simulink model "Torque Vectoring and Ackerman Model"  (R2020b)
settings: Solver=ode4  StartTime=0.0  StopTime=12  FixedStep=1e-5  RelTol=1e-3
InitFcn:
  | clc
  | clear
  | clc;
  | clear;
  | Ts=1e-5; %Sampling time
  | f=50; %Supply frequency
  | Rs=0.03553; %Stator resistance
  | Rr=0.02092; %Rotor resistance
  | Lls=0.000335; %Stator inductance
  | Llr=0.000335; %Rotor inductance
  | Lm=0.0151; %Mutual inductance
  | P=4; %Number of Poles
  | ts=(Lls+Lm)/Rs; % Stator time constant
  | Tr=(Llr+Lm)/Rr; % Rotor time constant
  | Ls=Lls+Lm;
  | Lrr=Llr+Lm;
  | J=1.25; %Inertia
  | F=0.03914; %Friction factor
  | VDC=580;
  | sigma=1-(Lm^2/(Ls*Lrr));
  | rs=Rs+Rr*(Lm/Lrr)^2;
  | Kp=1498*sigma*Ls;
  | Ki=rs*1498;
  | dw=1.55;
  | l=3;
  | m       =       1500;           %Vehicle mass
  | g       =       9.81;           %Gravitational acceleration
  | L       =          3;           %Distance between front axle and rear axle
  | Lf      =        1.3;           %Distance between center of mass and front axle
  | Lr      =       L-Lf;           %Distance between center of mass and rear axle
  | Cf      =      67369;           %Front track Cornering stiffness coef
  | Cr      =      63411;           %rear track Cornering stiffness coef
  | S       =        1.7;           %Area of frontal surface of the vehicle
  | CYB     =       -2.2;           %Force drag coef
  | CMzB    =        0.6;           %Moment drag coef
  | Mzfa    =       2010;           %Front track Aligning stiffness coef
  | Mzra    =       1366;           %rear track Aligning stiffness coef
  | rho     =      1.225;           %density
  | Iz      =       2000;           %Yaw Moment of Inertia
  | Kgear=1;
undefined symbols (not defined in the file): DiscIntNeverNeededParam, Driver, Wheels_Driver_VehDyn_Lib
libraries: pid_lib x12, powerlib_meascontrol x11, powerlib x9, simulink_extras x4
(part 2 of 2)

== system Torque Vectoring and Ackerman Model/Right Motor/FOC1/Vd ==
  Phir* : Inport
  id : Inport  Port=2
  Current PI : pid_lib/PID Controller  Controller=PI  Form=Parallel  TimeDomain=Discrete-time  UseExternalTs=off  SampleTime=Ts  IntegratorMethod=Forward Euler  FilterMethod=Forward Euler  ControllerParametersSource=internal  P=Kp  I=Ki  D=0  UseFilter=on  N=100  TunerSelectOption=Transfer Function Based (PID Tuner App)  InitialConditionSource=internal  InitialConditionForIntegrator=0  InitialConditionForFilter=0  DifferentiatorICPrevScaledInput=0  ExternalReset=none  TrackingMode=off  Kt=1  LimitOutput=on  SatLimitsSource=internal  UpperSaturationLimit=VDC  LowerSaturationLimit=-VDC/2  LinearizeAsGain=off  AntiWindupMode=clamping  Kb=1  POutMin=[]  POutMax=[]  IOutMin=[]  IOutMax=[]  DOutMin=[]  DOutMax=[]  NOutMin=[]  NOutMax=[]  SumOutMin=[]  SumOutMax=[]  SaturationOutMin=[]  SaturationOutMax=[]  PParamMin=[]  PParamMax=[]  IParamMin=[]  IParamMax=[]  DParamMin=[]  DParamMax=[]  NParamMin=[]  NParamMax=[]  KbParamMin=[]  KbParamMax=[]  KtParamMin=[]  KtParamMax=[]  KbOutMin=[]  KbOutMax=[]  KtOutMin=[]  KtOutMax=[]  IntegratorOutMin=[]  IntegratorOutMax=[]  FilterOutMin=[]  FilterOutMax=[]  SumI1OutMin=[]  SumI1OutMax=[]  SumI2OutMin=[]  SumI2OutMax=[]  SumI3OutMin=[]  SumI3OutMax=[]  SumI4OutMin=[]  SumI4OutMax=[]  SumDOutMin=[]  SumDOutMax=[]  DifferentiatorOutMin=[]  DifferentiatorOutMax=[]  FilterDiffOutCoefMin=[]  FilterDiffOutCoefMax=[]  ReciprocalOutMin=[]  ReciprocalOutMax=[]  SumDenOutMin=[]  SumDenOutMax=[]  SumNumOutMin=[]  SumNumOutMax=[]  DivideOutMin=[]  DivideOutMax=[]  UdiffTsProdOutMin=[]  UdiffTsProdOutMax=[]  NTsProdOutMin=[]  NTsProdOutMax=[]  UintegralTsProdOutMin=[]  UintegralTsProdOutMax=[]  UngainTsProdOutMin=[]  UngainTsProdOutMax=[]  IntegratorContinuousStateAttributes=''  IntegratorStateMustResolveToSignalObject=off  IntegratorRTWStateStorageClass=Auto  FilterContinuousStateAttributes=''  FilterStateMustResolveToSignalObject=off  FilterRTWStateStorageClass=Auto  ParallelPVariant=InternalParameters  IdealPVariant=Disabled  IVariant=InternalParameters  DVariant=Disabled  IntegratorVariant=Discrete  SatVariant=Enabled  AWVariant=DiscClampingParallel  PCopyVariant=Disabled  TRVariant=Disabled  FdbkBlocksVariant=Forward  IdealPFdbkVariant=Disabled  SatFdbkVariant=Disabled  DerivativeFilterVariant=Disabled  NVariant=Disabled  NCopyVariant=Disabled_SignalSpec  FilterICVariant=Disabled  IntegratorICVariant=InternalICs  ExternalResetVariant=Disabled  TRSumVariant=Passthrough  SumFdbkVariant=Disabled  SumVariant=Sum_PI  TsampFilterVariant=InternalTs  TsampNgainVariant=Passthrough  TsampIntegralVariant=Passthrough  ExternalSaturationOutDataTypeStr=Inherit: Same as second input
  Gain : Gain  Gain=1/Lm
  Scope : Scope
  Sum2 : Sum  Inputs=|+-
  Vd : Outport
  tag scope: IdrefR=global
  wires:
  Gain/1 -> [IdrefR], Scope/1, Sum2/1
  Phir*/1 -> Gain/1
  id/1 -> Sum2/2
  Sum2/1 -> Current PI/1
  Current PI/1 -> Vd/1

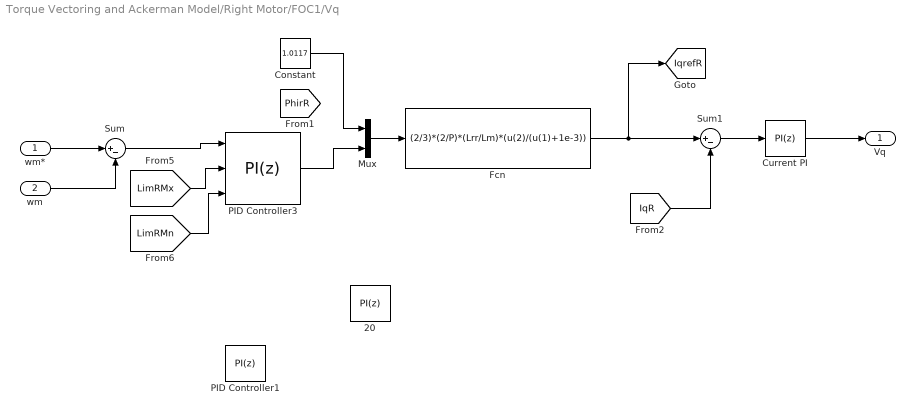
== system Torque Vectoring and Ackerman Model/Right Motor/FOC1/Vq ==
  wm* : Inport
  wm : Inport  Port=2
  20 : pid_lib/PID Controller  Controller=PI  Form=Parallel  TimeDomain=Discrete-time  UseExternalTs=off  SampleTime=-1  IntegratorMethod=Forward Euler  FilterMethod=Forward Euler  ControllerParametersSource=internal  P=152.4390244  I=9295.062463  D=0  UseFilter=on  N=100  TunerSelectOption=Transfer Function Based (PID Tuner App)  InitialConditionSource=internal  InitialConditionForIntegrator=0  InitialConditionForFilter=0  DifferentiatorICPrevScaledInput=0  ExternalReset=none  TrackingMode=off  Kt=1  LimitOutput=on  SatLimitsSource=internal  UpperSaturationLimit=960  LowerSaturationLimit=-960  LinearizeAsGain=off  AntiWindupMode=clamping  Kb=1  POutMin=[]  POutMax=[]  IOutMin=[]  IOutMax=[]  DOutMin=[]  DOutMax=[]  NOutMin=[]  NOutMax=[]  SumOutMin=[]  SumOutMax=[]  SaturationOutMin=[]  SaturationOutMax=[]  PParamMin=[]  PParamMax=[]  IParamMin=[]  IParamMax=[]  DParamMin=[]  DParamMax=[]  NParamMin=[]  NParamMax=[]  KbParamMin=[]  KbParamMax=[]  KtParamMin=[]  KtParamMax=[]  KbOutMin=[]  KbOutMax=[]  KtOutMin=[]  KtOutMax=[]  IntegratorOutMin=[]  IntegratorOutMax=[]  FilterOutMin=[]  FilterOutMax=[]  SumI1OutMin=[]  SumI1OutMax=[]  SumI2OutMin=[]  SumI2OutMax=[]  SumI3OutMin=[]  SumI3OutMax=[]  SumI4OutMin=[]  SumI4OutMax=[]  SumDOutMin=[]  SumDOutMax=[]  DifferentiatorOutMin=[]  DifferentiatorOutMax=[]  FilterDiffOutCoefMin=[]  FilterDiffOutCoefMax=[]  ReciprocalOutMin=[]  ReciprocalOutMax=[]  SumDenOutMin=[]  SumDenOutMax=[]  SumNumOutMin=[]  SumNumOutMax=[]  DivideOutMin=[]  DivideOutMax=[]  UdiffTsProdOutMin=[]  UdiffTsProdOutMax=[]  NTsProdOutMin=[]  NTsProdOutMax=[]  UintegralTsProdOutMin=[]  UintegralTsProdOutMax=[]  UngainTsProdOutMin=[]  UngainTsProdOutMax=[]  IntegratorContinuousStateAttributes=''  IntegratorStateMustResolveToSignalObject=off  IntegratorRTWStateStorageClass=Auto  FilterContinuousStateAttributes=''  FilterStateMustResolveToSignalObject=off  FilterRTWStateStorageClass=Auto  ParallelPVariant=InternalParameters  IdealPVariant=Disabled  IVariant=InternalParameters  DVariant=Disabled  IntegratorVariant=Discrete  SatVariant=Enabled  AWVariant=DiscClampingParallel  PCopyVariant=Disabled  TRVariant=Disabled  FdbkBlocksVariant=Forward  IdealPFdbkVariant=Disabled  SatFdbkVariant=Disabled  DerivativeFilterVariant=Disabled  NVariant=Disabled  NCopyVariant=Disabled_SignalSpec  FilterICVariant=Disabled  IntegratorICVariant=InternalICs  ExternalResetVariant=Disabled  TRSumVariant=Passthrough  SumFdbkVariant=Disabled  SumVariant=Sum_PI  TsampFilterVariant=InternalTs  TsampNgainVariant=Passthrough  TsampIntegralVariant=Passthrough  ExternalSaturationOutDataTypeStr=Inherit: Same as second input
  Constant : Constant  Value=1.0117
  Current PI : pid_lib/PID Controller  Controller=PI  Form=Parallel  TimeDomain=Discrete-time  UseExternalTs=off  SampleTime=Ts  IntegratorMethod=Forward Euler  FilterMethod=Forward Euler  ControllerParametersSource=internal  P=Kp  I=Ki  D=0  UseFilter=on  N=100  TunerSelectOption=Transfer Function Based (PID Tuner App)  InitialConditionSource=internal  InitialConditionForIntegrator=0  InitialConditionForFilter=0  DifferentiatorICPrevScaledInput=0  ExternalReset=none  TrackingMode=off  Kt=1  LimitOutput=on  SatLimitsSource=internal  UpperSaturationLimit=VDC/sqrt(3)  LowerSaturationLimit=-VDC/sqrt(3)  LinearizeAsGain=off  AntiWindupMode=clamping  Kb=1  POutMin=[]  POutMax=[]  IOutMin=[]  IOutMax=[]  DOutMin=[]  DOutMax=[]  NOutMin=[]  NOutMax=[]  SumOutMin=[]  SumOutMax=[]  SaturationOutMin=[]  SaturationOutMax=[]  PParamMin=[]  PParamMax=[]  IParamMin=[]  IParamMax=[]  DParamMin=[]  DParamMax=[]  NParamMin=[]  NParamMax=[]  KbParamMin=[]  KbParamMax=[]  KtParamMin=[]  KtParamMax=[]  KbOutMin=[]  KbOutMax=[]  KtOutMin=[]  KtOutMax=[]  IntegratorOutMin=[]  IntegratorOutMax=[]  FilterOutMin=[]  FilterOutMax=[]  SumI1OutMin=[]  SumI1OutMax=[]  SumI2OutMin=[]  SumI2OutMax=[]  SumI3OutMin=[]  SumI3OutMax=[]  SumI4OutMin=[]  SumI4OutMax=[]  SumDOutMin=[]  SumDOutMax=[]  DifferentiatorOutMin=[]  DifferentiatorOutMax=[]  FilterDiffOutCoefMin=[]  FilterDiffOutCoefMax=[]  ReciprocalOutMin=[]  ReciprocalOutMax=[]  SumDenOutMin=[]  SumDenOutMax=[]  SumNumOutMin=[]  SumNumOutMax=[]  DivideOutMin=[]  DivideOutMax=[]  UdiffTsProdOutMin=[]  UdiffTsProdOutMax=[]  NTsProdOutMin=[]  NTsProdOutMax=[]  UintegralTsProdOutMin=[]  UintegralTsProdOutMax=[]  UngainTsProdOutMin=[]  UngainTsProdOutMax=[]  IntegratorContinuousStateAttributes=''  IntegratorStateMustResolveToSignalObject=off  IntegratorRTWStateStorageClass=Auto  FilterContinuousStateAttributes=''  FilterStateMustResolveToSignalObject=off  FilterRTWStateStorageClass=Auto  ParallelPVariant=InternalParameters  IdealPVariant=Disabled  IVariant=InternalParameters  DVariant=Disabled  IntegratorVariant=Discrete  SatVariant=Enabled  AWVariant=DiscClampingParallel  PCopyVariant=Disabled  TRVariant=Disabled  FdbkBlocksVariant=Forward  IdealPFdbkVariant=Disabled  SatFdbkVariant=Disabled  DerivativeFilterVariant=Disabled  NVariant=Disabled  NCopyVariant=Disabled_SignalSpec  FilterICVariant=Disabled  IntegratorICVariant=InternalICs  ExternalResetVariant=Disabled  TRSumVariant=Passthrough  SumFdbkVariant=Disabled  SumVariant=Sum_PI  TsampFilterVariant=InternalTs  TsampNgainVariant=Passthrough  TsampIntegralVariant=Passthrough  ExternalSaturationOutDataTypeStr=Inherit: Same as second input
  Fcn : Fcn  Expr=(2/3)*(2/P)*(Lrr/Lm)*(u(2)/(u(1)+1e-3))
  Mux : Mux  Inputs=2
  PID Controller1 : pid_lib/PID Controller  Controller=PI  Form=Parallel  TimeDomain=Discrete-time  UseExternalTs=off  SampleTime=-1  IntegratorMethod=Forward Euler  FilterMethod=Forward Euler  ControllerParametersSource=internal  P=105.005210798555  I=869.041988278239  D=0  UseFilter=on  N=100  TunerSelectOption=Transfer Function Based (PID Tuner App)  InitialConditionSource=internal  InitialConditionForIntegrator=0  InitialConditionForFilter=0  DifferentiatorICPrevScaledInput=0  ExternalReset=none  TrackingMode=off  Kt=1  LimitOutput=on  SatLimitsSource=internal  UpperSaturationLimit=960  LowerSaturationLimit=-960  LinearizeAsGain=off  AntiWindupMode=clamping  Kb=1  POutMin=[]  POutMax=[]  IOutMin=[]  IOutMax=[]  DOutMin=[]  DOutMax=[]  NOutMin=[]  NOutMax=[]  SumOutMin=[]  SumOutMax=[]  SaturationOutMin=[]  SaturationOutMax=[]  PParamMin=[]  PParamMax=[]  IParamMin=[]  IParamMax=[]  DParamMin=[]  DParamMax=[]  NParamMin=[]  NParamMax=[]  KbParamMin=[]  KbParamMax=[]  KtParamMin=[]  KtParamMax=[]  KbOutMin=[]  KbOutMax=[]  KtOutMin=[]  KtOutMax=[]  IntegratorOutMin=[]  IntegratorOutMax=[]  FilterOutMin=[]  FilterOutMax=[]  SumI1OutMin=[]  SumI1OutMax=[]  SumI2OutMin=[]  SumI2OutMax=[]  SumI3OutMin=[]  SumI3OutMax=[]  SumI4OutMin=[]  SumI4OutMax=[]  SumDOutMin=[]  SumDOutMax=[]  DifferentiatorOutMin=[]  DifferentiatorOutMax=[]  FilterDiffOutCoefMin=[]  FilterDiffOutCoefMax=[]  ReciprocalOutMin=[]  ReciprocalOutMax=[]  SumDenOutMin=[]  SumDenOutMax=[]  SumNumOutMin=[]  SumNumOutMax=[]  DivideOutMin=[]  DivideOutMax=[]  UdiffTsProdOutMin=[]  UdiffTsProdOutMax=[]  NTsProdOutMin=[]  NTsProdOutMax=[]  UintegralTsProdOutMin=[]  UintegralTsProdOutMax=[]  UngainTsProdOutMin=[]  UngainTsProdOutMax=[]  IntegratorContinuousStateAttributes=''  IntegratorStateMustResolveToSignalObject=off  IntegratorRTWStateStorageClass=Auto  FilterContinuousStateAttributes=''  FilterStateMustResolveToSignalObject=off  FilterRTWStateStorageClass=Auto  ParallelPVariant=InternalParameters  IdealPVariant=Disabled  IVariant=InternalParameters  DVariant=Disabled  IntegratorVariant=Discrete  SatVariant=Enabled  AWVariant=DiscClampingParallel  PCopyVariant=Disabled  TRVariant=Disabled  FdbkBlocksVariant=Forward  IdealPFdbkVariant=Disabled  SatFdbkVariant=Disabled  DerivativeFilterVariant=Disabled  NVariant=Disabled  NCopyVariant=Disabled_SignalSpec  FilterICVariant=Disabled  IntegratorICVariant=InternalICs  ExternalResetVariant=Disabled  TRSumVariant=Passthrough  SumFdbkVariant=Disabled  SumVariant=Sum_PI  TsampFilterVariant=InternalTs  TsampNgainVariant=Passthrough  TsampIntegralVariant=Passthrough  ExternalSaturationOutDataTypeStr=Inherit: Same as second input
  PID Controller3 : pid_lib/PID Controller  Controller=PI  Form=Parallel  TimeDomain=Discrete-time  UseExternalTs=off  SampleTime=-1  IntegratorMethod=Forward Euler  FilterMethod=Forward Euler  ControllerParametersSource=internal  P=152.4390244  I=9295.062463  D=0  UseFilter=on  N=100  TunerSelectOption=Transfer Function Based (PID Tuner App)  InitialConditionSource=internal  InitialConditionForIntegrator=0  InitialConditionForFilter=0  DifferentiatorICPrevScaledInput=0  ExternalReset=none  TrackingMode=off  Kt=1  LimitOutput=on  SatLimitsSource=external  UpperSaturationLimit=960  LowerSaturationLimit=-960  LinearizeAsGain=off  AntiWindupMode=clamping  Kb=1  POutMin=[]  POutMax=[]  IOutMin=[]  IOutMax=[]  DOutMin=[]  DOutMax=[]  NOutMin=[]  NOutMax=[]  SumOutMin=[]  SumOutMax=[]  SaturationOutMin=[]  SaturationOutMax=[]  PParamMin=[]  PParamMax=[]  IParamMin=[]  IParamMax=[]  DParamMin=[]  DParamMax=[]  NParamMin=[]  NParamMax=[]  KbParamMin=[]  KbParamMax=[]  KtParamMin=[]  KtParamMax=[]  KbOutMin=[]  KbOutMax=[]  KtOutMin=[]  KtOutMax=[]  IntegratorOutMin=[]  IntegratorOutMax=[]  FilterOutMin=[]  FilterOutMax=[]  SumI1OutMin=[]  SumI1OutMax=[]  SumI2OutMin=[]  SumI2OutMax=[]  SumI3OutMin=[]  SumI3OutMax=[]  SumI4OutMin=[]  SumI4OutMax=[]  SumDOutMin=[]  SumDOutMax=[]  DifferentiatorOutMin=[]  DifferentiatorOutMax=[]  FilterDiffOutCoefMin=[]  FilterDiffOutCoefMax=[]  ReciprocalOutMin=[]  ReciprocalOutMax=[]  SumDenOutMin=[]  SumDenOutMax=[]  SumNumOutMin=[]  SumNumOutMax=[]  DivideOutMin=[]  DivideOutMax=[]  UdiffTsProdOutMin=[]  UdiffTsProdOutMax=[]  NTsProdOutMin=[]  NTsProdOutMax=[]  UintegralTsProdOutMin=[]  UintegralTsProdOutMax=[]  UngainTsProdOutMin=[]  UngainTsProdOutMax=[]  IntegratorContinuousStateAttributes=''  IntegratorStateMustResolveToSignalObject=off  IntegratorRTWStateStorageClass=Auto  FilterContinuousStateAttributes=''  FilterStateMustResolveToSignalObject=off  FilterRTWStateStorageClass=Auto  ParallelPVariant=InternalParameters  IdealPVariant=Disabled  IVariant=InternalParameters  DVariant=Disabled  IntegratorVariant=Discrete  SatVariant=External  AWVariant=DiscClampingParallel  PCopyVariant=Disabled  TRVariant=Disabled  FdbkBlocksVariant=Forward  IdealPFdbkVariant=Disabled  SatFdbkVariant=Disabled  DerivativeFilterVariant=Disabled  NVariant=Disabled  NCopyVariant=Disabled_SignalSpec  FilterICVariant=Disabled  IntegratorICVariant=InternalICs  ExternalResetVariant=Disabled  TRSumVariant=Passthrough  SumFdbkVariant=Disabled  SumVariant=Sum_PI  TsampFilterVariant=InternalTs  TsampNgainVariant=Passthrough  TsampIntegralVariant=Passthrough  ExternalSaturationOutDataTypeStr=Inherit: Same as second input
  Sum : Sum  Inputs=|+-
  Sum1 : Sum  Inputs=|+-
  Vq : Outport
  tag scope: IqrefR=global
  wires:
  wm/1 -> Sum/2
  Mux/1 -> Fcn/1
  wm*/1 -> Sum/1
  [IqR] -> Sum1/2
  Fcn/1 -> Sum1/1, [IqrefR]
  Sum1/1 -> Current PI/1
  Current PI/1 -> Vq/1
  Constant/1 -> Mux/1
  Sum/1 -> PID Controller3/1
  PID Controller3/1 -> Mux/2
  [LimRMx] -> PID Controller3/2
  [LimRMn] -> PID Controller3/3

== matlab function Torque Vectoring and Ackerman Model/Adjustment/MATLAB Function1 ==
  data: WmR input; LimRMx output; WmL input; LimRMn output; Tl input; LimLMx output; LimLMn output
function [LimRMx, LimRMn, LimLMx, LimLMn]= fcn(WmR,WmL,Tl)
LimMx = 960;
LimMn = -960;
    LimRMx = LimMx;
    LimRMn = LimMn;
    LimLMx = LimMx;
    LimLMn = LimMn;    
if WmR > WmL
    LimRMx = LimMx;
    LimLMn = -(LimRMx-Tl)+Tl;
    LimRMn = -(LimRMx-Tl)+Tl;
    LimLMx = LimMx;
elseif WmR < WmL
     LimLMx = LimMx;
     LimRMn = - (LimLMx-Tl)+Tl;
     LimLMn=- (LimLMx-Tl)+Tl;
     LimRMx=LimMx;
end
end

== matlab function Torque Vectoring and Ackerman Model/Toruqe Vectoring/CorrectionModel/MATLAB Function2 ==
  data: dT output; delta input; V input; Mze output; beta input; YawRate input; Tleft output; Tright output; TorqueLoad input
function [dT,Mze,Tleft,Tright] = fcn(delta, V, beta, YawRate,TorqueLoad)
m       =       1500;           %Vehicle mass
g       =       9.81;           %Gravitational acceleration
L       =          3;           %Distance between front axle and rear axle
Lf      =        1.3;           %Distance between center of mass and front axle
Lr      =       L-Lf;           %Distance between center of mass and rear axle
Cf      =      67369;           %Front track Cornering stiffness coef
Cr      =      63411;           %rear track Cornering stiffness coef
S       =        1.7;           %Area of frontal surface of the vehicle 
CYB     =       -2.2;           %Force drag coef
CMzB    =        0.6;           %Moment drag coef
Mzfa    =       2010;           %Front track Aligning stiffness coef
Mzra    =       1366;           %rear track Aligning stiffness coef
rho     =      1.225;           %density
Iz      =       2000;           %Yaw Moment of Inertia
WR      =       0.3;
W       =       1.56;
%Drivatives of stability for lateral forces
Ybeta   =                 -(Cf + Cr + 0.5* rho * V^2 * S * CYB);
Yr      =                                -(1/V)*(Lf*Cf - Lr*Cr);
Ydelta  =                                                    Cf;
%Derivatives of stability for Yawing moment
Nbeta   =   (-Lf*Cf + Lr*Cr + Mzfa + Mzra) + 0.5*rho*V^2*S*CMzB;
Nr      =         (1/V)*(-Lf^2*Cf - Lr^2*Cr+ Mzfa*Lf - Mzra*Lr);
Ndelta  =                                         Cf*Lf - Mzfa ;
%Dynamic Matrix
A       =   [Ybeta/(m*V), (Yr/(m*V)-1);
               Nbeta/Iz, Nr / (Iz)    ];
%Input Gain Matrix 
B       =           [Ydelta/(m*V);
                      Ndelta/Iz  ];
%Linearized behaviour &mass-spring-damper analogy
P       =                           V*Iz*m;   %Mass
Q       =                 -Ybeta*Iz-V*m*Nr;   %Damping Coef
U       =        Nbeta*(V*m-Yr) + Nr*Ybeta;   %Stiffness

Sd      =      -Ndelta*(V*m-Yr)-Nr*Ydelta;
Sdd     =     Ydelta*Nbeta - Ndelta*Ybeta;
Td      =                       Iz*Ydelta;
Tdd     =                      V*m*Ndelta;
ddelta  =                               0;
Fye     =                               0;
Mzedot  =                               0;
rdot    =                               0;
if delta == 0
    Mze = 0;   
else
    Mze     = ((Sdd*delta + Tdd*ddelta + Nbeta*Fye + m*V*Mzedot - Q*rdot - U*YawRate)/Ybeta)/4;
end
Treq =  TorqueLoad/4;
dT = Mze*WR/W;
Tleft =Treq-dT;
Tright=Treq+dT;
Bc =[0;Mze/Iz];
